simulink model "CostasLoop"  (R2025b)
settings: Solver=VariableStepAuto  StartTime=0.0  StopTime=2  RelTol=1e-3
undefined symbols (not defined in the file): dspblkCoreblockFVToolHelper, gcbh, h
libraries: dspsigops x1
settings Model: Creator=sakha  LastModifiedBy=sakha

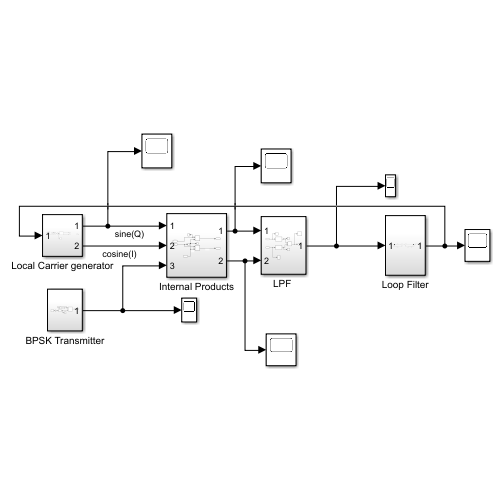
[thumbnail: Simulink's stored preview of the top-level diagram]
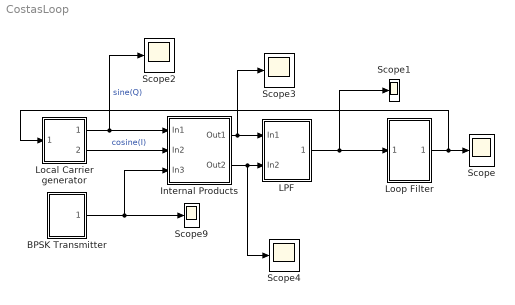
== system CostasLoop ==
  BPSK Transmitter : Subsystem
  Internal Products : Subsystem
  "LPF " : Subsystem
  Local Carrier generator : Subsystem
  Loop Filter : Subsystem
  Scope{,1..4,9} (6 alike) : Scope
      Scope settings: ActiveDisplayYMinimum=-0.00054518519195247248  ActiveDisplayYMaximum=0.0008701967317078749  DataLoggingVariableName=output
      Scope1 settings: ActiveDisplayYMinimum=-0.080839117240954259  ActiveDisplayYMaximum=0.23777350572652434  DataLoggingVariableName=ScopeData5
      Scope2 settings: ActiveDisplayYMinimum=-0.70246587424679086  ActiveDisplayYMaximum=0.49937442862257359  DataLoggingVariableName=ScopeData15
      Scope3 settings: ActiveDisplayYMinimum=-2.706109942780238  ActiveDisplayYMaximum=4.9995815686098251  DataLoggingVariableName=ScopeData16
      Scope4 settings: ActiveDisplayYMinimum=-1.1888156100342389  ActiveDisplayYMaximum=1.1888200858873084  DataLoggingVariableName=ScopeData17
      Scope9 settings: ActiveDisplayYMinimum=-1.1888206453689421  ActiveDisplayYMaximum=1.1888206453689421  DataLoggingVariableName=ScopeData9
  wires:
  BPSK Transmitter/1(Out1) -> Scope9/1, Internal Products/3(In3)
  Local Carrier generator/1(Out1) -> Scope2/1, Internal Products/1(In1)  "sine(Q)"
  Local Carrier generator/2(Out2) -> Internal Products/2(In2)  "cosine(I)"
  Internal Products/1(Out1) -> Scope3/1, "LPF "/1(In1)
  Internal Products/2(Out2) -> Scope4/1, "LPF "/2(In2)
  Loop Filter/1(Out2) -> Local Carrier generator/1(In1), Scope/1
  "LPF "/1(Out1) -> Scope1/1, Loop Filter/1(In1)

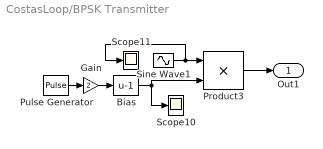
== system CostasLoop/BPSK Transmitter ==
  Bias : Bias  Bias=-1  SaturateOnIntegerOverflow=off
  Gain : Gain  Gain=2
  Product3 : Product
  Pulse Generator : DiscretePulseGenerator  Period=320  PulseWidth=160  SampleTime=1.5625e-6
  Scope10 : Scope
      settings: DataLoggingVariableName=ScopeData10
  Scope11 : Scope
      settings: ActiveDisplayYMinimum=-1.3366675243834765  ActiveDisplayYMaximum=1.9487858924253851  DataLoggingVariableName=ScopeData11
  Sine Wave1 : Sin  SineType=Sample based  SampleTime=1.5625e-6
  Out1 : Outport
  wires:
  Pulse Generator/1 -> Gain/1
  Sine Wave1/1 -> Scope11/1, Product3/1
  Bias/1 -> Scope10/1, Product3/2
  Gain/1 -> Bias/1
  Product3/1 -> Out1/1

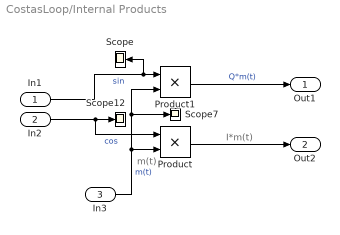
== system CostasLoop/Internal Products ==
  note: I*m(t)
  note: m(t)
  In1 : Inport
  In2 : Inport  Port=2
  In3 : Inport  Port=3
  Product : Product
  Product1 : Product
  Scope : Scope
      settings: ActiveDisplayYMinimum=-1  ActiveDisplayYMaximum=1  DataLoggingVariableName=ScopeData8
  Scope12 : Scope
      settings: ActiveDisplayYMinimum=-4.4291141879237443  ActiveDisplayYMaximum=8.7439942512439526  DataLoggingVariableName=ScopeData12
  Scope7 : Scope
      settings: ActiveDisplayYMinimum=-1.4039748697863019  ActiveDisplayYMaximum=3.6329366796809395  DataLoggingVariableName=ScopeData7
  Out1 : Outport
  Out2 : Outport  Port=2
  wires:
  In2/1 -> Product/1, Scope12/1  "cos"
  In3/1 -> Scope7/1, Product1/2, Product/2  "m(t)"
  In1/1 -> Product1/1, Scope/1  "sin"
  Product1/1 -> Out1/1  "Q*m(t)"
  Product/1 -> Out2/1

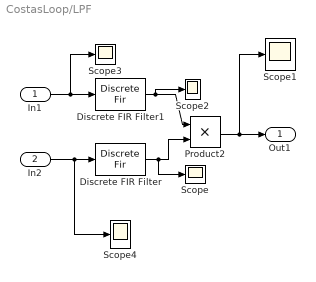
== system CostasLoop/LPF  ==
  In1 : Inport
  In2 : Inport  Port=2
  Discrete FIR Filter : DiscreteFir  LoadFcn=dspblkCoreblockFVToolHelper(gcbh,'load');  Coefficients=h  InputProcessing=Columns as channels (frame based)
      settings: CopyFcn=dspblkCoreblockFVToolHelper(gcbh,'copy');  DeleteFcn=dspblkCoreblockFVToolHelper(gcbh,'close');  ModelCloseFcn=dspblkCoreblockFVToolHelper(gcbh,'close');  PreSaveFcn=dspblkCoreblockFVToolHelper(gcbh,'presave');  PostSaveFcn=dspblkCoreblockFVToolHelper(gcbh,'postsave');  CloseFcn=dspblkCoreblockFVToolHelper(gcbh,'close');
  Discrete FIR Filter1 : DiscreteFir  LoadFcn=dspblkCoreblockFVToolHelper(gcbh,'load');  Coefficients=h  InputProcessing=Columns as channels (frame based)
      settings: CopyFcn=dspblkCoreblockFVToolHelper(gcbh,'copy');  DeleteFcn=dspblkCoreblockFVToolHelper(gcbh,'close');  ModelCloseFcn=dspblkCoreblockFVToolHelper(gcbh,'close');  PreSaveFcn=dspblkCoreblockFVToolHelper(gcbh,'presave');  PostSaveFcn=dspblkCoreblockFVToolHelper(gcbh,'postsave');  CloseFcn=dspblkCoreblockFVToolHelper(gcbh,'close');
  Product2 : Product
  Scope{,1..4} (5 alike) : Scope
      Scope settings: ActiveDisplayYMinimum=-0.81516529188454  ActiveDisplayYMaximum=0.57930064276306
      Scope1 settings: ActiveDisplayYMinimum=-0.29898721533919703  ActiveDisplayYMaximum=0.48476572654186068  DataLoggingVariableName=ScopeData14
      Scope2 settings: ActiveDisplayYMinimum=-0.62503006687511864  ActiveDisplayYMaximum=0.62503567173600294  DataLoggingVariableName=ScopeData2
      Scope3 settings: ActiveDisplayYMinimum=-1.2935848696606589  ActiveDisplayYMaximum=1.2816655387975746  DataLoggingVariableName=ScopeData3
      Scope4 settings: ActiveDisplayYMinimum=-1.5727800846772582  ActiveDisplayYMaximum=1.5917015357127429  DataLoggingVariableName=ScopeData4
  Out1 : Outport
  wires:
  Discrete FIR Filter/1 -> Scope/1, Product2/2
  In2/1 -> Scope4/1, Discrete FIR Filter/1
  Discrete FIR Filter1/1 -> Scope2/1, Product2/1
  In1/1 -> Scope3/1, Discrete FIR Filter1/1
  Product2/1 -> Scope1/1, Out1/1

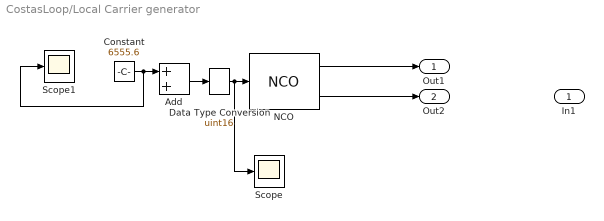
== system CostasLoop/Local Carrier generator ==
  In1 : Inport
  Add : Sum
  Constant : Constant  Value=6555.6
  Data Type Conversion : DataTypeConversion  OutDataTypeStr=uint16  SaturateOnIntegerOverflow=off  RndMeth=Floor
  NCO : dspsigops/NCO  AccIncSrc=Input port  AccInc=100  PhaseOffsetSrc=Specify via dialog  PhaseOffset=0  AccumWL=17  HasDither=off  DitherWL=4  PNgeneratorLength=19  HasPhaseQuantizer=on  TableDepth=16  HasOutputPhaseError=off  Formula=Sine and cosine  DataType=double  OutputWL=16  OutputFL=14  CompMethod=Table lookup (no interpolation)  SampleTime=1  SamplesPerFrame=1  OutputFrames=off
  Scope : Scope
      settings: ActiveDisplayYMinimum=5501.2892004753412  ActiveDisplayYMaximum=7795.84840035496  DataLoggingVariableName=ScopeData6
  Scope1 : Scope
      settings: ActiveDisplayYMinimum=5568.4641529935261  ActiveDisplayYMaximum=7538.0428684161006  DataLoggingVariableName=ScopeData13
  Out1 : Outport
  Out2 : Outport  Port=2
  wires:
  NCO/2 -> Out2/1
  Add/1 -> Data Type Conversion/1
  NCO/1 -> Out1/1
  Data Type Conversion/1 -> Scope/1, NCO/1
  Constant/1 -> Scope1/1, Add/1

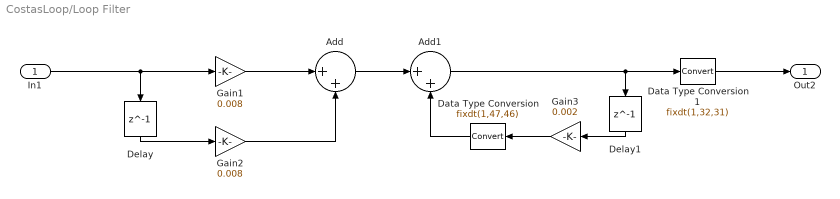
== system CostasLoop/Loop Filter ==
  In1 : Inport
  Add : Sum  Inputs=|++  OutDataTypeStr=fixdt(1,47,46)  AccumDataTypeStr=fixdt(1,47,46)
  Add1 : Sum  Inputs=|++  OutDataTypeStr=fixdt(1,47,46)  AccumDataTypeStr=fixdt(1,47,46)
  Data Type Conversion : DataTypeConversion  OutDataTypeStr=fixdt(1,47,46)  SaturateOnIntegerOverflow=off  RndMeth=Floor
  Data Type Conversion1 : DataTypeConversion  OutDataTypeStr=fixdt(1,32,31)  SaturateOnIntegerOverflow=off  RndMeth=Floor
  Delay : Delay  DelayLength=1  InitialCondition=0
  Delay1 : Delay  DelayLength=1  InitialCondition=0
  Gain1 : Gain  Gain=0.008  ParamDataTypeStr=fixdt(1,32,31)  OutDataTypeStr=fixdt(1,47,46)
  Gain2 : Gain  Gain=0.008  ParamDataTypeStr=fixdt(1,32,31)  OutDataTypeStr=fixdt(1,47,46)
  Gain3 : Gain  Gain=0.002  ParamDataTypeStr=fixdt(1,32,31)  OutDataTypeStr=fixdt(1,79,78)
  Out2 : Outport
  wires:
  Delay/1 -> Gain2/1
  Gain1/1 -> Add/1
  Add1/1 -> Delay1/1, Data Type Conversion1/1
  Gain2/1 -> Add/2
  Data Type Conversion/1 -> Add1/2
  Delay1/1 -> Gain3/1
  Data Type Conversion1/1 -> Out2/1
  In1/1 -> Gain1/1, Delay/1
  Add/1 -> Add1/1
  Gain3/1 -> Data Type Conversion/1
